simulink model "EV_Modelling"  (R2023b)
settings: Solver=VariableStepAuto  StartTime=0.0  StopTime=500  RelTol=1e-3
libraries: simulink x1
settings Model: Creator=HP5CD  LastModifiedBy=HP5CD

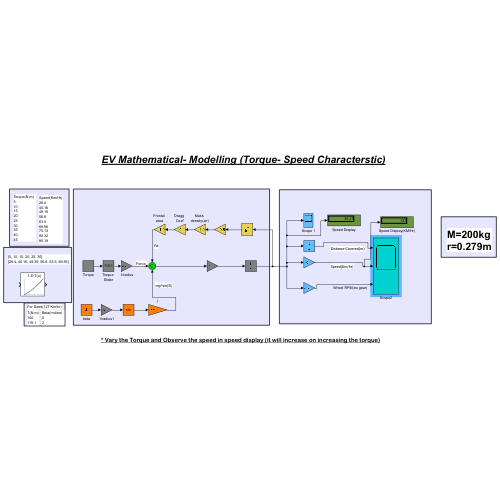
[thumbnail: Simulink's stored preview of the top-level diagram]
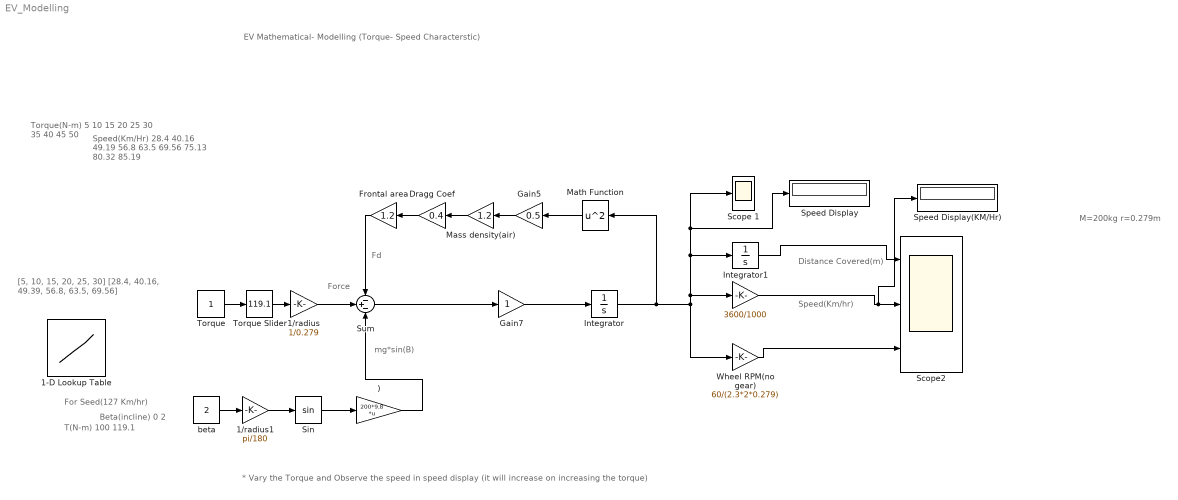
== system EV_Modelling ==
  note: Force
  note: [5, 10, 15, 20, 25, 30]
      | [28.4, 40.16, 49.39, 56.8, 63.5, 69.56]
  note: For Seed(127 Km/hr)
  note: Beta(incline)
      | 0
      | 2
  note: T(N-m)
      | 100
      | 119.1
  note: Speed(Km/Hr)
      | 28.4
      | 40.16
      | 49.19
      | 56.8
      | 63.5
      | 69.56
      | 75.13
      | 80.32
      | 85.19
  note: Torque(N-m)
      | 5
      | 10
      | 15
      | 20
      | 25
      | 30
      | 35
      | 40
      | 45
      | 50
  note: M=200kg
      | r=0.279m
  note: * Vary the Torque and Observe the speed in speed display (it will increase on increasing the torque)
  note: EV Mathematical- Modelling (Torque- Speed Characterstic)
  note: mg*sin(B)
  note: Fd
  note: Speed(Km/hr)
  note: Distance Covered(m)
  "                " : Gain  Gain=3600/1000
  "                Wheel RPM(no gear)" : Gain  Gain=60/(2.3*2*0.279)
  ) : Gain  Gain=200*9.8  Multiplication=Matrix(K*u)
  1-D Lookup Table : Lookup_n-D  NumberOfTableDimensions=1  BreakpointsForDimension1=[28.4, 40.16, 49.39, 56.8, 63.5, 69.56]  Table=[5, 10, 15, 20, 25, 30]  InternalRulePriority=Speed  RndMeth=Simplest
  1/radius : Gain  Gain=1/0.279
  1/radius1 : Gain  Gain=pi/180
  Dragg Coef : Gain  Gain=0.4
  Frontal area : Gain  Gain=1.2
  Gain5 : Gain  Gain=0.5
  Gain7 : Gain
  Integrator : Integrator
  Integrator1 : Integrator
  Mass density(air) : Gain  Gain=1.2
  Math Function : Math  Operator=square
  Scope 1 : Scope
  Scope2 : Scope  NumInputPorts=3
  Sin : Trigonometry
  Speed Display : Display
  Speed Display(KM/Hr) : Display
  Sum : Sum  Inputs=-+-
  Torque : Constant
  Torque Slider : simulink/Math Operations/Slider Gain  gain=119.1  low=1  high=200
  beta : Constant  Value=2
  wires:
  Dragg Coef/1 -> Frontal area/1
  Gain5/1 -> Mass density(air)/1
  Mass density(air)/1 -> Dragg Coef/1
  Torque/1 -> Torque Slider/1
  1/radius/1 -> Sum/2
  Gain7/1 -> Integrator/1
  Sum/1 -> Gain7/1
  Math Function/1 -> Gain5/1
  Frontal area/1 -> Sum/1
  Integrator/1 -> Integrator1/1, Speed Display/1, Scope 1/1, "                "/1, "                Wheel RPM(no gear)"/1, Math Function/1
  Sin/1 -> )/1
  )/1 -> Sum/3
  beta/1 -> 1/radius1/1
  Integrator1/1 -> Scope2/1
  "                "/1 -> Speed Display(KM/Hr)/1, Scope2/2
  "                Wheel RPM(no gear)"/1 -> Scope2/3
  1/radius1/1 -> Sin/1
  Torque Slider/1 -> 1/radius/1
